simulink model "Demo_MostImportant_cs"  (R2014b)
settings: Solver=FixedStepDiscrete  SolverMode=SingleTasking  StartTime=0.0  StopTime=18  FixedStep=1/20  RelTol=1e-3
PreLoadFcn:
  | mbxruntime.callbacks.PreLoadFcn(bdroot);
  | check_NUTS_defined
  | model_closed = 0;
  | assignin('base',['model_closed_' bdroot],false);
PostLoadFcn:
  | mbxruntime.callbacks.PostLoadFcn(bdroot);
InitFcn:
  | mbxruntime.callbacks.InitFcn(bdroot);
StartFcn:
  | mbxruntime.callbacks.StartFcn(bdroot);
StopFcn:
  | mbxruntime.callbacks.StopFcn(bdroot);;
  | 
model workspace: external: MAT-File .\Demo_MostImportant_cs_hws.mat (data not in the file)
undefined symbols (not defined in the file or in its folder): mbxruntime, tabledata
undefined symbols (not defined in the file): Demo_MostImportant_cs_05200168a21c2533, Demo_MostImportant_cs_094a97935dc182a0, Demo_MostImportant_cs_0f0a9e0d54ccafda, Demo_MostImportant_cs_0fd3352235f3d862, Demo_MostImportant_cs_143c6c4f39bdc546, Demo_MostImportant_cs_20660bde6631f89a, Demo_MostImportant_cs_22077597b1c7a4aa, Demo_MostImportant_cs_22569723bd476150, Demo_MostImportant_cs_25eb058b93ed81ed, Demo_MostImportant_cs_27ad505fd49d0562, Demo_MostImportant_cs_3388db03542917da, Demo_MostImportant_cs_3411dde5ae0dc98c, Demo_MostImportant_cs_365f965ea4b6cb52, Demo_MostImportant_cs_3bee97dace5a3f8a, Demo_MostImportant_cs_3d2ef73ad714ff29, Demo_MostImportant_cs_4312029ae1b23d3a, Demo_MostImportant_cs_431f249e57fff8cb, Demo_MostImportant_cs_437388c3dfd4518f, Demo_MostImportant_cs_439f7e889f94edbe, Demo_MostImportant_cs_44a44174db621f6d, Demo_MostImportant_cs_4a7f7efcfc625194, Demo_MostImportant_cs_4a85c22e4a955f8e, Demo_MostImportant_cs_4c0e276e17a8ce88, Demo_MostImportant_cs_4cf092a47043b63b, Demo_MostImportant_cs_528dc6b548c718e3, Demo_MostImportant_cs_554a5828426d1258, Demo_MostImportant_cs_5a7163d13d0d3a72, Demo_MostImportant_cs_5d58a9d5d373adee, Demo_MostImportant_cs_60fd2791e6a88e66, Demo_MostImportant_cs_62ee6b3874c5d210, Demo_MostImportant_cs_63cb394815d07d4b, Demo_MostImportant_cs_660ed07c6769932e, Demo_MostImportant_cs_704620a5d39b7df9, Demo_MostImportant_cs_715ca1aaa17d3e85, Demo_MostImportant_cs_72b0848bf20979d6, Demo_MostImportant_cs_786125b10b06ee8f, Demo_MostImportant_cs_7e81a3b41a2b3c89, Demo_MostImportant_cs_81a32c4ed1a9050c, Demo_MostImportant_cs_883a94dece8b903d, Demo_MostImportant_cs_90ff3a0811121d4c, Demo_MostImportant_cs_912cf0a5d0300393, Demo_MostImportant_cs_99d08ec3ace083e5, Demo_MostImportant_cs_9be8f6a6d15b97ae, Demo_MostImportant_cs_a1434df4461c57cd, Demo_MostImportant_cs_a9807fe959845dbd, Demo_MostImportant_cs_ad42817c2f688b9e, Demo_MostImportant_cs_Audi_A8_2_Path_pathUniqueID, Demo_MostImportant_cs_b5f63321977d4686, Demo_MostImportant_cs_bae02335aafbc09b, Demo_MostImportant_cs_bdb138340502b82e, Demo_MostImportant_cs_be891ccddc71916a, Demo_MostImportant_cs_BMW_X5_1_Path_pathUniqueID, Demo_MostImportant_cs_BMW_X5_2_Path_pathUniqueID, Demo_MostImportant_cs_c0dcb6f642224268, Demo_MostImportant_cs_c311fdddc66ce1e1, Demo_MostImportant_cs_c34fad1f7dbabd44, Demo_MostImportant_cs_c3ed80f4b140c4cf, Demo_MostImportant_cs_c71d57cd5d2ef8b2, Demo_MostImportant_cs_Citroen_C3_2_Path_pathUniqueID, Demo_MostImportant_cs_d6fc18532502b855 ... (+12)
libraries: PreScanSimulinkLibrary x20, simulink x16, PreScanUsefulBlocks x1
(part 4 of 7)

== system Demo_MostImportant_cs/VISUColorRegion_Exterior_Audi_A8_1 ==
  VISUColorRegion_Exterior_Audi_A8_1 : Inport  Tag=inport/ColorRegion  OutDataTypeStr=Bus: PRESCAN_COLOR_DATA  PortDimensions=1  SampleTime=1/20  BusOutputAsStruct=on
  Actuator : S-Function  FunctionName=sfun_ColorActuator  Parameters=mbxruntime.parameters.convert(UniqueID), mbxruntime.parameters.convert(WorldModelSubPath),tabledata, TimeStep  EnableBusSupport=off  mask(PreScan Sink Block: VisuTextureColor){UniqueID=49, WorldModelSubPath=/recolorRegion:name=Exterior/targetColor, TimeStep=1/20}
      mask prompts: UniqueID "Parent Unique Identifier (auto-generated)"; WorldModelSubPath "WM SubPath(auto-generated)"; TimeStep "Simulink time step"
      mask help:
      | The VisuTextureColor block provides a way to adapt the color of a vehicle.
      |
      | For more information, please click Help.
      mask init:
      | [tabledata] = mbxruntime.parameters.table(UniqueID,WorldModelSubPath);
      mask Help: eval('openHelp(230)')
      mask Display: image(imread('TextureColor.png'))
  wires:
  VISUColorRegion_Exterior_Audi_A8_1/1 -> Actuator/1

== system Demo_MostImportant_cs/VISUColorRegion_Exterior_Audi_A8_2 ==
  VISUColorRegion_Exterior_Audi_A8_2 : Inport  Tag=inport/ColorRegion  OutDataTypeStr=Bus: PRESCAN_COLOR_DATA  PortDimensions=1  SampleTime=1/20  BusOutputAsStruct=on
  Actuator : S-Function  FunctionName=sfun_ColorActuator  Parameters=mbxruntime.parameters.convert(UniqueID), mbxruntime.parameters.convert(WorldModelSubPath),tabledata, TimeStep  EnableBusSupport=off  mask(PreScan Sink Block: VisuTextureColor){UniqueID=107, WorldModelSubPath=/recolorRegion:name=Exterior/targetColor, TimeStep=1/20}
      mask prompts: UniqueID "Parent Unique Identifier (auto-generated)"; WorldModelSubPath "WM SubPath(auto-generated)"; TimeStep "Simulink time step"
      mask help:
      | The VisuTextureColor block provides a way to adapt the color of a vehicle.
      |
      | For more information, please click Help.
      mask init:
      | [tabledata] = mbxruntime.parameters.table(UniqueID,WorldModelSubPath);
      mask Help: eval('openHelp(230)')
      mask Display: image(imread('TextureColor.png'))
  wires:
  VISUColorRegion_Exterior_Audi_A8_2/1 -> Actuator/1

== system Demo_MostImportant_cs/VISUColorRegion_Exterior_Audi_A8_3 ==
  VISUColorRegion_Exterior_Audi_A8_3 : Inport  Tag=inport/ColorRegion  OutDataTypeStr=Bus: PRESCAN_COLOR_DATA  PortDimensions=1  SampleTime=1/20  BusOutputAsStruct=on
  Actuator : S-Function  FunctionName=sfun_ColorActuator  Parameters=mbxruntime.parameters.convert(UniqueID), mbxruntime.parameters.convert(WorldModelSubPath),tabledata, TimeStep  EnableBusSupport=off  mask(PreScan Sink Block: VisuTextureColor){UniqueID=143, WorldModelSubPath=/recolorRegion:name=Exterior/targetColor, TimeStep=1/20}
      mask prompts: UniqueID "Parent Unique Identifier (auto-generated)"; WorldModelSubPath "WM SubPath(auto-generated)"; TimeStep "Simulink time step"
      mask help:
      | The VisuTextureColor block provides a way to adapt the color of a vehicle.
      |
      | For more information, please click Help.
      mask init:
      | [tabledata] = mbxruntime.parameters.table(UniqueID,WorldModelSubPath);
      mask Help: eval('openHelp(230)')
      mask Display: image(imread('TextureColor.png'))
  wires:
  VISUColorRegion_Exterior_Audi_A8_3/1 -> Actuator/1

== system Demo_MostImportant_cs/VISUColorRegion_Exterior_BMW_X5_1 ==
  VISUColorRegion_Exterior_BMW_X5_1 : Inport  Tag=inport/ColorRegion  OutDataTypeStr=Bus: PRESCAN_COLOR_DATA  PortDimensions=1  SampleTime=1/20  BusOutputAsStruct=on
  Actuator : S-Function  FunctionName=sfun_ColorActuator  Parameters=mbxruntime.parameters.convert(UniqueID), mbxruntime.parameters.convert(WorldModelSubPath),tabledata, TimeStep  EnableBusSupport=off  mask(PreScan Sink Block: VisuTextureColor){UniqueID=19, WorldModelSubPath=/recolorRegion:name=Exterior/targetColor, TimeStep=1/20}
      mask prompts: UniqueID "Parent Unique Identifier (auto-generated)"; WorldModelSubPath "WM SubPath(auto-generated)"; TimeStep "Simulink time step"
      mask help:
      | The VisuTextureColor block provides a way to adapt the color of a vehicle.
      |
      | For more information, please click Help.
      mask init:
      | [tabledata] = mbxruntime.parameters.table(UniqueID,WorldModelSubPath);
      mask Help: eval('openHelp(230)')
      mask Display: image(imread('TextureColor.png'))
  wires:
  VISUColorRegion_Exterior_BMW_X5_1/1 -> Actuator/1

== system Demo_MostImportant_cs/VISUColorRegion_Exterior_BMW_X5_2 ==
  VISUColorRegion_Exterior_BMW_X5_2 : Inport  Tag=inport/ColorRegion  OutDataTypeStr=Bus: PRESCAN_COLOR_DATA  PortDimensions=1  SampleTime=1/20  BusOutputAsStruct=on
  Actuator : S-Function  FunctionName=sfun_ColorActuator  Parameters=mbxruntime.parameters.convert(UniqueID), mbxruntime.parameters.convert(WorldModelSubPath),tabledata, TimeStep  EnableBusSupport=off  mask(PreScan Sink Block: VisuTextureColor){UniqueID=111, WorldModelSubPath=/recolorRegion:name=Exterior/targetColor, TimeStep=1/20}
      mask prompts: UniqueID "Parent Unique Identifier (auto-generated)"; WorldModelSubPath "WM SubPath(auto-generated)"; TimeStep "Simulink time step"
      mask help:
      | The VisuTextureColor block provides a way to adapt the color of a vehicle.
      |
      | For more information, please click Help.
      mask init:
      | [tabledata] = mbxruntime.parameters.table(UniqueID,WorldModelSubPath);
      mask Help: eval('openHelp(230)')
      mask Display: image(imread('TextureColor.png'))
  wires:
  VISUColorRegion_Exterior_BMW_X5_2/1 -> Actuator/1

== system Demo_MostImportant_cs/VISUColorRegion_Exterior_Citroen_C3_1 ==
  VISUColorRegion_Exterior_Citroen_C3_1 : Inport  Tag=inport/ColorRegion  OutDataTypeStr=Bus: PRESCAN_COLOR_DATA  PortDimensions=1  SampleTime=1/20  BusOutputAsStruct=on
  Actuator : S-Function  FunctionName=sfun_ColorActuator  Parameters=mbxruntime.parameters.convert(UniqueID), mbxruntime.parameters.convert(WorldModelSubPath),tabledata, TimeStep  EnableBusSupport=off  mask(PreScan Sink Block: VisuTextureColor){UniqueID=45, WorldModelSubPath=/recolorRegion:name=Exterior/targetColor, TimeStep=1/20}
      mask prompts: UniqueID "Parent Unique Identifier (auto-generated)"; WorldModelSubPath "WM SubPath(auto-generated)"; TimeStep "Simulink time step"
      mask help:
      | The VisuTextureColor block provides a way to adapt the color of a vehicle.
      |
      | For more information, please click Help.
      mask init:
      | [tabledata] = mbxruntime.parameters.table(UniqueID,WorldModelSubPath);
      mask Help: eval('openHelp(230)')
      mask Display: image(imread('TextureColor.png'))
  wires:
  VISUColorRegion_Exterior_Citroen_C3_1/1 -> Actuator/1

== system Demo_MostImportant_cs/VISUColorRegion_Exterior_Citroen_C3_2 ==
  VISUColorRegion_Exterior_Citroen_C3_2 : Inport  Tag=inport/ColorRegion  OutDataTypeStr=Bus: PRESCAN_COLOR_DATA  PortDimensions=1  SampleTime=1/20  BusOutputAsStruct=on
  Actuator : S-Function  FunctionName=sfun_ColorActuator  Parameters=mbxruntime.parameters.convert(UniqueID), mbxruntime.parameters.convert(WorldModelSubPath),tabledata, TimeStep  EnableBusSupport=off  mask(PreScan Sink Block: VisuTextureColor){UniqueID=117, WorldModelSubPath=/recolorRegion:name=Exterior/targetColor, TimeStep=1/20}
      mask prompts: UniqueID "Parent Unique Identifier (auto-generated)"; WorldModelSubPath "WM SubPath(auto-generated)"; TimeStep "Simulink time step"
      mask help:
      | The VisuTextureColor block provides a way to adapt the color of a vehicle.
      |
      | For more information, please click Help.
      mask init:
      | [tabledata] = mbxruntime.parameters.table(UniqueID,WorldModelSubPath);
      mask Help: eval('openHelp(230)')
      mask Display: image(imread('TextureColor.png'))
  wires:
  VISUColorRegion_Exterior_Citroen_C3_2/1 -> Actuator/1

== system Demo_MostImportant_cs/VISUColorRegion_Exterior_Citroen_C3_3 ==
  VISUColorRegion_Exterior_Citroen_C3_3 : Inport  Tag=inport/ColorRegion  OutDataTypeStr=Bus: PRESCAN_COLOR_DATA  PortDimensions=1  SampleTime=1/20  BusOutputAsStruct=on
  Actuator : S-Function  FunctionName=sfun_ColorActuator  Parameters=mbxruntime.parameters.convert(UniqueID), mbxruntime.parameters.convert(WorldModelSubPath),tabledata, TimeStep  EnableBusSupport=off  mask(PreScan Sink Block: VisuTextureColor){UniqueID=139, WorldModelSubPath=/recolorRegion:name=Exterior/targetColor, TimeStep=1/20}
      mask prompts: UniqueID "Parent Unique Identifier (auto-generated)"; WorldModelSubPath "WM SubPath(auto-generated)"; TimeStep "Simulink time step"
      mask help:
      | The VisuTextureColor block provides a way to adapt the color of a vehicle.
      |
      | For more information, please click Help.
      mask init:
      | [tabledata] = mbxruntime.parameters.table(UniqueID,WorldModelSubPath);
      mask Help: eval('openHelp(230)')
      mask Display: image(imread('TextureColor.png'))
  wires:
  VISUColorRegion_Exterior_Citroen_C3_3/1 -> Actuator/1

== system Demo_MostImportant_cs/VISUColorRegion_Exterior_Citroen_C3_4 ==
  VISUColorRegion_Exterior_Citroen_C3_4 : Inport  Tag=inport/ColorRegion  OutDataTypeStr=Bus: PRESCAN_COLOR_DATA  PortDimensions=1  SampleTime=1/20  BusOutputAsStruct=on
  Actuator : S-Function  FunctionName=sfun_ColorActuator  Parameters=mbxruntime.parameters.convert(UniqueID), mbxruntime.parameters.convert(WorldModelSubPath),tabledata, TimeStep  EnableBusSupport=off  mask(PreScan Sink Block: VisuTextureColor){UniqueID=140, WorldModelSubPath=/recolorRegion:name=Exterior/targetColor, TimeStep=1/20}
      mask prompts: UniqueID "Parent Unique Identifier (auto-generated)"; WorldModelSubPath "WM SubPath(auto-generated)"; TimeStep "Simulink time step"
      mask help:
      | The VisuTextureColor block provides a way to adapt the color of a vehicle.
      |
      | For more information, please click Help.
      mask init:
      | [tabledata] = mbxruntime.parameters.table(UniqueID,WorldModelSubPath);
      mask Help: eval('openHelp(230)')
      mask Display: image(imread('TextureColor.png'))
  wires:
  VISUColorRegion_Exterior_Citroen_C3_4/1 -> Actuator/1

== system Demo_MostImportant_cs/VISUColorRegion_Exterior_Toyota_Previa_1 ==
  VISUColorRegion_Exterior_Toyota_Previa_1 : Inport  Tag=inport/ColorRegion  OutDataTypeStr=Bus: PRESCAN_COLOR_DATA  PortDimensions=1  SampleTime=1/20  BusOutputAsStruct=on
  Actuator : S-Function  FunctionName=sfun_ColorActuator  Parameters=mbxruntime.parameters.convert(UniqueID), mbxruntime.parameters.convert(WorldModelSubPath),tabledata, TimeStep  EnableBusSupport=off  mask(PreScan Sink Block: VisuTextureColor){UniqueID=15, WorldModelSubPath=/recolorRegion:name=Exterior/targetColor, TimeStep=1/20}
      mask prompts: UniqueID "Parent Unique Identifier (auto-generated)"; WorldModelSubPath "WM SubPath(auto-generated)"; TimeStep "Simulink time step"
      mask help:
      | The VisuTextureColor block provides a way to adapt the color of a vehicle.
      |
      | For more information, please click Help.
      mask init:
      | [tabledata] = mbxruntime.parameters.table(UniqueID,WorldModelSubPath);
      mask Help: eval('openHelp(230)')
      mask Display: image(imread('TextureColor.png'))
  wires:
  VISUColorRegion_Exterior_Toyota_Previa_1/1 -> Actuator/1

== system Demo_MostImportant_cs/VISUColorRegion_Exterior_Toyota_Previa_2 ==
  VISUColorRegion_Exterior_Toyota_Previa_2 : Inport  Tag=inport/ColorRegion  OutDataTypeStr=Bus: PRESCAN_COLOR_DATA  PortDimensions=1  SampleTime=1/20  BusOutputAsStruct=on
  Actuator : S-Function  FunctionName=sfun_ColorActuator  Parameters=mbxruntime.parameters.convert(UniqueID), mbxruntime.parameters.convert(WorldModelSubPath),tabledata, TimeStep  EnableBusSupport=off  mask(PreScan Sink Block: VisuTextureColor){UniqueID=99, WorldModelSubPath=/recolorRegion:name=Exterior/targetColor, TimeStep=1/20}
      mask prompts: UniqueID "Parent Unique Identifier (auto-generated)"; WorldModelSubPath "WM SubPath(auto-generated)"; TimeStep "Simulink time step"
      mask help:
      | The VisuTextureColor block provides a way to adapt the color of a vehicle.
      |
      | For more information, please click Help.
      mask init:
      | [tabledata] = mbxruntime.parameters.table(UniqueID,WorldModelSubPath);
      mask Help: eval('openHelp(230)')
      mask Display: image(imread('TextureColor.png'))
  wires:
  VISUColorRegion_Exterior_Toyota_Previa_2/1 -> Actuator/1

== system Demo_MostImportant_cs/VISUColorRegion_Exterior_Toyota_Previa_3 ==
  VISUColorRegion_Exterior_Toyota_Previa_3 : Inport  Tag=inport/ColorRegion  OutDataTypeStr=Bus: PRESCAN_COLOR_DATA  PortDimensions=1  SampleTime=1/20  BusOutputAsStruct=on
  Actuator : S-Function  FunctionName=sfun_ColorActuator  Parameters=mbxruntime.parameters.convert(UniqueID), mbxruntime.parameters.convert(WorldModelSubPath),tabledata, TimeStep  EnableBusSupport=off  mask(PreScan Sink Block: VisuTextureColor){UniqueID=123, WorldModelSubPath=/recolorRegion:name=Exterior/targetColor, TimeStep=1/20}
      mask prompts: UniqueID "Parent Unique Identifier (auto-generated)"; WorldModelSubPath "WM SubPath(auto-generated)"; TimeStep "Simulink time step"
      mask help:
      | The VisuTextureColor block provides a way to adapt the color of a vehicle.
      |
      | For more information, please click Help.
      mask init:
      | [tabledata] = mbxruntime.parameters.table(UniqueID,WorldModelSubPath);
      mask Help: eval('openHelp(230)')
      mask Display: image(imread('TextureColor.png'))
  wires:
  VISUColorRegion_Exterior_Toyota_Previa_3/1 -> Actuator/1

== system Demo_MostImportant_cs/VISUColorRegion_Exterior_Toyota_Previa_4 ==
  VISUColorRegion_Exterior_Toyota_Previa_4 : Inport  Tag=inport/ColorRegion  OutDataTypeStr=Bus: PRESCAN_COLOR_DATA  PortDimensions=1  SampleTime=1/20  BusOutputAsStruct=on
  Actuator : S-Function  FunctionName=sfun_ColorActuator  Parameters=mbxruntime.parameters.convert(UniqueID), mbxruntime.parameters.convert(WorldModelSubPath),tabledata, TimeStep  EnableBusSupport=off  mask(PreScan Sink Block: VisuTextureColor){UniqueID=141, WorldModelSubPath=/recolorRegion:name=Exterior/targetColor, TimeStep=1/20}
      mask prompts: UniqueID "Parent Unique Identifier (auto-generated)"; WorldModelSubPath "WM SubPath(auto-generated)"; TimeStep "Simulink time step"
      mask help:
      | The VisuTextureColor block provides a way to adapt the color of a vehicle.
      |
      | For more information, please click Help.
      mask init:
      | [tabledata] = mbxruntime.parameters.table(UniqueID,WorldModelSubPath);
      mask Help: eval('openHelp(230)')
      mask Display: image(imread('TextureColor.png'))
  wires:
  VISUColorRegion_Exterior_Toyota_Previa_4/1 -> Actuator/1

== system Demo_MostImportant_cs/VISUColorRegion_Exterior_Toyota_Yaris_1 ==
  VISUColorRegion_Exterior_Toyota_Yaris_1 : Inport  Tag=inport/ColorRegion  OutDataTypeStr=Bus: PRESCAN_COLOR_DATA  PortDimensions=1  SampleTime=1/20  BusOutputAsStruct=on
  Actuator : S-Function  FunctionName=sfun_ColorActuator  Parameters=mbxruntime.parameters.convert(UniqueID), mbxruntime.parameters.convert(WorldModelSubPath),tabledata, TimeStep  EnableBusSupport=off  mask(PreScan Sink Block: VisuTextureColor){UniqueID=46, WorldModelSubPath=/recolorRegion:name=Exterior/targetColor, TimeStep=1/20}
      mask prompts: UniqueID "Parent Unique Identifier (auto-generated)"; WorldModelSubPath "WM SubPath(auto-generated)"; TimeStep "Simulink time step"
      mask help:
      | The VisuTextureColor block provides a way to adapt the color of a vehicle.
      |
      | For more information, please click Help.
      mask init:
      | [tabledata] = mbxruntime.parameters.table(UniqueID,WorldModelSubPath);
      mask Help: eval('openHelp(230)')
      mask Display: image(imread('TextureColor.png'))
  wires:
  VISUColorRegion_Exterior_Toyota_Yaris_1/1 -> Actuator/1

== system Demo_MostImportant_cs/VISUColorRegion_Exterior_Toyota_Yaris_2 ==
  VISUColorRegion_Exterior_Toyota_Yaris_2 : Inport  Tag=inport/ColorRegion  OutDataTypeStr=Bus: PRESCAN_COLOR_DATA  PortDimensions=1  SampleTime=1/20  BusOutputAsStruct=on
  Actuator : S-Function  FunctionName=sfun_ColorActuator  Parameters=mbxruntime.parameters.convert(UniqueID), mbxruntime.parameters.convert(WorldModelSubPath),tabledata, TimeStep  EnableBusSupport=off  mask(PreScan Sink Block: VisuTextureColor){UniqueID=142, WorldModelSubPath=/recolorRegion:name=Exterior/targetColor, TimeStep=1/20}
      mask prompts: UniqueID "Parent Unique Identifier (auto-generated)"; WorldModelSubPath "WM SubPath(auto-generated)"; TimeStep "Simulink time step"
      mask help:
      | The VisuTextureColor block provides a way to adapt the color of a vehicle.
      |
      | For more information, please click Help.
      mask init:
      | [tabledata] = mbxruntime.parameters.table(UniqueID,WorldModelSubPath);
      mask Help: eval('openHelp(230)')
      mask Display: image(imread('TextureColor.png'))
  wires:
  VISUColorRegion_Exterior_Toyota_Yaris_2/1 -> Actuator/1

== system Demo_MostImportant_cs/Audi_A8_1/Dynamics_Empty ==
  note: For state mode 'Dynamic' positions
      | are not taken into account, as they
      | are computed by integrating velocity.
      | Click annotation for Help.
  Ground_{1..9} (9 alike) : Ground
  MuxState : Subsystem  Tag=mux/State  mask(Empty Dynamics State Block){positioningmode=on, TimeStep=1/20}
      mask prompts: positioningmode "Positioning Mode"; TimeStep "Auto Assigned: Time Step [s]"
      mask help:
      | Build the state of an actor based on user input.
      | The user can either use positioning mode or dynamics mode.
      | - When using positioning mode the position and orientation of the actor are set directly based on the input. Expected input is relative to the initial position and orientation of the actor. It's also possible to specify the velocity of the actor, though this input isn't used, only passed on.
      | - When using dynamics mode the position input is ignored. Expected input is velocity and orientation. The velocity is relative the current orientation of the actor, while orientation is relative to its initial orientation. The position of the actor is calculated based on the velocity and orientation given.
      settings: DeleteFcn=PreScanBlockDeleteFcn;
  STATE_Audi_A8_1 : Subsystem  Tag=mux/StatePort  Priority=0  LoadFcn=load PrescanStateActuatorData  mask(PreScan Sink Block: State){x0=Demo_MostImportant_cs_df769faa31fd9ead, y0=Demo_MostImportant_cs_f67437bd412fea32, z0=Demo_MostImportant_cs_f04d43c825bf3ceb, Roll0=Demo_MostImportant_cs_3411dde5ae0dc98c, Pitch0=Demo_MostImportant_cs_5d58a9d5d373adee, Yaw0=Demo_MostImportant_cs_554a5828426d1258, TimeStep=1/20}
      mask prompts: x0 "Ini x-position VEHICLE wrt GLOBAL axis system [m]"; y0 "Ini y-position VEHICLE wrt GLOBAL axis system [m]"; z0 "Ini z-position VEHICLE wrt GLOBAL axis system [m]"; Roll0 "Ini roll-angle BODY wrt VEHICLE axis system [deg]"; Pitch0 "Ini pitch-angle BODY wrt VEHICLE axis system [deg]"; Yaw0 "Ini yaw-angle VEHICLE wrt GLOBAL axis system [deg]"; TimeStep "Auto-Assigned: Upload Period [s]"
      mask help:
      | The Actor State contains a vector signal of size (9x1), containing the following signals:
      |
      | -  Position                  (x,y,z)                                     [m]
      | -  Velocity                  (vx,vy,vz)                               [m/s]
      | -  Angles                    (Roll, Pitch, Yaw)                   [rad]
      |
      | The Actor state is defined in the global axis system.
      | The state is superponed on the Initial position defined in the GUI.
      |
      | For more information, please click Help.
      settings: DeleteFcn=PreScanBlockDeleteFcn;
      mask Help: eval('openHelp(222)')
      mask Display: image(imread('State.png'))
  State : Outport  Tag=outport/StateOutport  SampleTime=1/20
  wires:
  MuxState/1(state) -> STATE_Audi_A8_1/1(State)
  STATE_Audi_A8_1/1(StateBus) -> State/1
  Ground_1/1 -> MuxState/1(x [m])
  Ground_2/1 -> MuxState/2(y [m])
  Ground_3/1 -> MuxState/3(z [m])
  Ground_4/1 -> MuxState/4(dx [m/s])
  Ground_5/1 -> MuxState/5(dy [m/s])
  Ground_6/1 -> MuxState/6(dz [m/s])
  Ground_7/1 -> MuxState/7(R [rad])
  Ground_8/1 -> MuxState/8(P [rad])
  Ground_9/1 -> MuxState/9(Y [rad])

== system Demo_MostImportant_cs/Audi_A8_1/SELF_Demux ==
  SELF : Inport  OutDataTypeStr=Bus: PRESCAN_SELFSENSORDATA
  Bus Selector : BusSelector  OutputSignals=PositionX,PositionY,PositionZ,OrientationRoll,OrientationPitch,OrientationYaw,Velocity,Yaw_rate,Lat,Long,Alt
  Demux2 : Demux  Outputs=3
  Gain : Gain  Gain=180/pi
  Gain1 : Gain  Gain=180/pi
  Vector Concatenate1 : Concatenate  NumInputs=3
  compas converter : Subsystem
  x [m] : Outport
  y [m] : Outport  Port=2
  z [m] : Outport  Port=3
  rotx [deg] : Outport  Port=4
  roty [deg] : Outport  Port=5
  rotz [deg] : Outport  Port=6
  GPS lat [deg] : Outport  Port=7
  GPS long [deg] : Outport  Port=8
  GPS alt [m] : Outport  Port=9
  velocity [m/s] : Outport  Port=10
  heading [deg] : Outport  Port=11
  yaw rate [deg/s] : Outport  Port=12
  wires:
  Bus Selector/11 -> GPS alt [m]/1  "<Alt>"
  Bus Selector/10 -> GPS long [deg]/1  "<Long>"
  Bus Selector/9 -> GPS lat [deg]/1  "<Lat>"
  Bus Selector/8 -> Gain1/1  "<Yaw_rate>"
  Bus Selector/7 -> velocity [m/s]/1  "<Velocity>"
  Bus Selector/6 -> compas converter/1(rotz [rad]), Vector Concatenate1/3  "<OrientationYaw>"
  Bus Selector/5 -> Vector Concatenate1/2  "<OrientationPitch>"
  Bus Selector/4 -> Vector Concatenate1/1  "<OrientationRoll>"
  Vector Concatenate1/1 -> Gain/1
  Bus Selector/3 -> z [m]/1  "<PositionZ>"
  Bus Selector/2 -> y [m]/1  "<PositionY>"
  Bus Selector/1 -> x [m]/1  "<PositionX>"
  SELF/1 -> Bus Selector/1
  Gain/1 -> Demux2/1
  Demux2/1 -> rotx [deg]/1
  Demux2/2 -> roty [deg]/1
  Demux2/3 -> rotz [deg]/1
  compas converter/1(heading [deg]) -> heading [deg]/1
  Gain1/1 -> yaw rate [deg/s]/1

== system Demo_MostImportant_cs/Audi_A8_1/VISUColorRegion_Exterior_Mux ==
  RGB [-,-,-] : Inport
  Bus Creator : BusCreator  OutDataTypeStr=Bus: PRESCAN_COLOR_DATA  NonVirtualBus=on
  Constant : Constant  Value=255  OutDataTypeStr=uint8
  Data Type Conversion : DataTypeConversion  OutDataTypeStr=uint8
  Data Type Conversion1 : DataTypeConversion  OutDataTypeStr=uint8
  Data Type Conversion2 : DataTypeConversion  OutDataTypeStr=uint8
  Demux : Demux  Outputs=3
  ColorRegion : Outport  OutDataTypeStr=Bus: PRESCAN_COLOR_DATA  PortDimensions=1
  wires:
  Constant/1 -> Bus Creator/4  "A"
  Data Type Conversion2/1 -> Bus Creator/3  "B"
  Data Type Conversion1/1 -> Bus Creator/2  "G"
  Data Type Conversion/1 -> Bus Creator/1  "R"
  Demux/3 -> Data Type Conversion2/1  "B"
  Demux/2 -> Data Type Conversion1/1  "G"
  Demux/1 -> Data Type Conversion/1  "R"
  RGB [-,-,-]/1 -> Demux/1
  Bus Creator/1 -> ColorRegion/1

== system Demo_MostImportant_cs/Audi_A8_1/color_changing_logic ==
  Index_order : Inport
  Compare To Constant : simulink/Logic and Bit Operations/Compare To Constant  relop=<=  const=3  OutDataTypeStr=uint8  ZeroCross=off
  Multiport Switch : MultiPortSwitch  DataPortOrder=Zero-based contiguous  Inputs=4  zeroidx=on
  Product : Product  RndMeth=Zero
  TextureColor1 : Constant  Tag=TextureColor  Value="[255 0  0]"
  TextureColor2 : Constant  Tag=TextureColor  Value="[211  211  211]"
  TextureColor3 : Constant  Tag=TextureColor  Value=[255 128 0]
  TextureColor4 : Constant  Tag=TextureColor  Value=[255 255 55]
  RGB : Outport
  wires:
  TextureColor2/1 -> Multiport Switch/2  "L21"
  TextureColor1/1 -> Multiport Switch/3  "L21"
  TextureColor3/1 -> Multiport Switch/4
  Compare To Constant/1 -> Product/2
  Index_order/1 -> Product/1, Compare To Constant/1
  Product/1 -> Multiport Switch/1
  Multiport Switch/1 -> RGB/1  "L47"
  TextureColor4/1 -> Multiport Switch/5

== system Demo_MostImportant_cs/Audi_A8_2/SELF_Demux ==
  SELF : Inport  OutDataTypeStr=Bus: PRESCAN_SELFSENSORDATA
  Bus Selector : BusSelector  OutputSignals=PositionX,PositionY,PositionZ,OrientationRoll,OrientationPitch,OrientationYaw,Velocity,Yaw_rate,Lat,Long,Alt
  Demux2 : Demux  Outputs=3
  Gain : Gain  Gain=180/pi
  Gain1 : Gain  Gain=180/pi
  Vector Concatenate1 : Concatenate  NumInputs=3
  compas converter : Subsystem
  x [m] : Outport
  y [m] : Outport  Port=2
  z [m] : Outport  Port=3
  rotx [deg] : Outport  Port=4
  roty [deg] : Outport  Port=5
  rotz [deg] : Outport  Port=6
  GPS lat [deg] : Outport  Port=7
  GPS long [deg] : Outport  Port=8
  GPS alt [m] : Outport  Port=9
  velocity [m/s] : Outport  Port=10
  heading [deg] : Outport  Port=11
  yaw rate [deg/s] : Outport  Port=12
  wires:
  Bus Selector/11 -> GPS alt [m]/1  "<Alt>"
  Bus Selector/10 -> GPS long [deg]/1  "<Long>"
  Bus Selector/9 -> GPS lat [deg]/1  "<Lat>"
  Bus Selector/8 -> Gain1/1  "<Yaw_rate>"
  Bus Selector/7 -> velocity [m/s]/1  "<Velocity>"
  Bus Selector/6 -> compas converter/1(rotz [rad]), Vector Concatenate1/3  "<OrientationYaw>"
  Bus Selector/5 -> Vector Concatenate1/2  "<OrientationPitch>"
  Bus Selector/4 -> Vector Concatenate1/1  "<OrientationRoll>"
  Vector Concatenate1/1 -> Gain/1
  Bus Selector/3 -> z [m]/1  "<PositionZ>"
  Bus Selector/2 -> y [m]/1  "<PositionY>"
  Bus Selector/1 -> x [m]/1  "<PositionX>"
  SELF/1 -> Bus Selector/1
  Gain/1 -> Demux2/1
  Demux2/1 -> rotx [deg]/1
  Demux2/2 -> roty [deg]/1
  Demux2/3 -> rotz [deg]/1
  compas converter/1(heading [deg]) -> heading [deg]/1
  Gain1/1 -> yaw rate [deg/s]/1

== system Demo_MostImportant_cs/Audi_A8_2/VISUColorRegion_Exterior_Mux ==
  RGB [-,-,-] : Inport
  Bus Creator : BusCreator  OutDataTypeStr=Bus: PRESCAN_COLOR_DATA  NonVirtualBus=on
  Constant : Constant  Value=255  OutDataTypeStr=uint8
  Data Type Conversion : DataTypeConversion  OutDataTypeStr=uint8
  Data Type Conversion1 : DataTypeConversion  OutDataTypeStr=uint8
  Data Type Conversion2 : DataTypeConversion  OutDataTypeStr=uint8
  Demux : Demux  Outputs=3
  ColorRegion : Outport  OutDataTypeStr=Bus: PRESCAN_COLOR_DATA  PortDimensions=1
  wires:
  Constant/1 -> Bus Creator/4  "A"
  Data Type Conversion2/1 -> Bus Creator/3  "B"
  Data Type Conversion1/1 -> Bus Creator/2  "G"
  Data Type Conversion/1 -> Bus Creator/1  "R"
  Demux/3 -> Data Type Conversion2/1  "B"
  Demux/2 -> Data Type Conversion1/1  "G"
  Demux/1 -> Data Type Conversion/1  "R"
  RGB [-,-,-]/1 -> Demux/1
  Bus Creator/1 -> ColorRegion/1

== system Demo_MostImportant_cs/Audi_A8_2/color_changing_logic ==
  Index_order : Inport
  Compare To Constant : simulink/Logic and Bit Operations/Compare To Constant  relop=<=  const=3  OutDataTypeStr=uint8  ZeroCross=off
  Multiport Switch : MultiPortSwitch  DataPortOrder=Zero-based contiguous  Inputs=4  zeroidx=on
  Product : Product  RndMeth=Zero
  TextureColor1 : Constant  Tag=TextureColor  Value="[255 0  0]"
  TextureColor2 : Constant  Tag=TextureColor  Value="[211  211  211]"
  TextureColor3 : Constant  Tag=TextureColor  Value=[255 128 0]
  TextureColor4 : Constant  Tag=TextureColor  Value=[255 255 55]
  RGB : Outport
  wires:
  TextureColor2/1 -> Multiport Switch/2  "L21"
  TextureColor1/1 -> Multiport Switch/3  "L21"
  TextureColor3/1 -> Multiport Switch/4
  Compare To Constant/1 -> Product/2
  Index_order/1 -> Product/1, Compare To Constant/1
  Product/1 -> Multiport Switch/1
  Multiport Switch/1 -> RGB/1  "L47"
  TextureColor4/1 -> Multiport Switch/5

== system Demo_MostImportant_cs/Audi_A8_3/Dynamics_Empty ==
  note: For state mode 'Dynamic' positions
      | are not taken into account, as they
      | are computed by integrating velocity.
      | Click annotation for Help.
  Ground_{1..9} (9 alike) : Ground
  MuxState : Subsystem  Tag=mux/State  mask(Empty Dynamics State Block){positioningmode=on, TimeStep=1/20}
      mask prompts: positioningmode "Positioning Mode"; TimeStep "Auto Assigned: Time Step [s]"
      mask help:
      | Build the state of an actor based on user input.
      | The user can either use positioning mode or dynamics mode.
      | - When using positioning mode the position and orientation of the actor are set directly based on the input. Expected input is relative to the initial position and orientation of the actor. It's also possible to specify the velocity of the actor, though this input isn't used, only passed on.
      | - When using dynamics mode the position input is ignored. Expected input is velocity and orientation. The velocity is relative the current orientation of the actor, while orientation is relative to its initial orientation. The position of the actor is calculated based on the velocity and orientation given.
      settings: DeleteFcn=PreScanBlockDeleteFcn;
  STATE_Audi_A8_3 : Subsystem  Tag=mux/StatePort  Priority=0  LoadFcn=load PrescanStateActuatorData  mask(PreScan Sink Block: State){x0=Demo_MostImportant_cs_ad42817c2f688b9e, y0=Demo_MostImportant_cs_4312029ae1b23d3a, z0=Demo_MostImportant_cs_a9807fe959845dbd, Roll0=Demo_MostImportant_cs_365f965ea4b6cb52, Pitch0=Demo_MostImportant_cs_3388db03542917da, Yaw0=Demo_MostImportant_cs_05200168a21c2533, TimeStep=1/20}
      mask prompts: x0 "Ini x-position VEHICLE wrt GLOBAL axis system [m]"; y0 "Ini y-position VEHICLE wrt GLOBAL axis system [m]"; z0 "Ini z-position VEHICLE wrt GLOBAL axis system [m]"; Roll0 "Ini roll-angle BODY wrt VEHICLE axis system [deg]"; Pitch0 "Ini pitch-angle BODY wrt VEHICLE axis system [deg]"; Yaw0 "Ini yaw-angle VEHICLE wrt GLOBAL axis system [deg]"; TimeStep "Auto-Assigned: Upload Period [s]"
      mask help:
      | The Actor State contains a vector signal of size (9x1), containing the following signals:
      |
      | -  Position                  (x,y,z)                                     [m]
      | -  Velocity                  (vx,vy,vz)                               [m/s]
      | -  Angles                    (Roll, Pitch, Yaw)                   [rad]
      |
      | The Actor state is defined in the global axis system.
      | The state is superponed on the Initial position defined in the GUI.
      |
      | For more information, please click Help.
      settings: DeleteFcn=PreScanBlockDeleteFcn;
      mask Help: eval('openHelp(222)')
      mask Display: image(imread('State.png'))
  State : Outport  Tag=outport/StateOutport  SampleTime=1/20
  wires:
  MuxState/1(state) -> STATE_Audi_A8_3/1(State)
  STATE_Audi_A8_3/1(StateBus) -> State/1
  Ground_1/1 -> MuxState/1(x [m])
  Ground_2/1 -> MuxState/2(y [m])
  Ground_3/1 -> MuxState/3(z [m])
  Ground_4/1 -> MuxState/4(dx [m/s])
  Ground_5/1 -> MuxState/5(dy [m/s])
  Ground_6/1 -> MuxState/6(dz [m/s])
  Ground_7/1 -> MuxState/7(R [rad])
  Ground_8/1 -> MuxState/8(P [rad])
  Ground_9/1 -> MuxState/9(Y [rad])

== system Demo_MostImportant_cs/Audi_A8_3/SELF_Demux ==
  SELF : Inport  OutDataTypeStr=Bus: PRESCAN_SELFSENSORDATA
  Bus Selector : BusSelector  OutputSignals=PositionX,PositionY,PositionZ,OrientationRoll,OrientationPitch,OrientationYaw,Velocity,Yaw_rate,Lat,Long,Alt
  Demux2 : Demux  Outputs=3
  Gain : Gain  Gain=180/pi
  Gain1 : Gain  Gain=180/pi
  Vector Concatenate1 : Concatenate  NumInputs=3
  compas converter : Subsystem
  x [m] : Outport
  y [m] : Outport  Port=2
  z [m] : Outport  Port=3
  rotx [deg] : Outport  Port=4
  roty [deg] : Outport  Port=5
  rotz [deg] : Outport  Port=6
  GPS lat [deg] : Outport  Port=7
  GPS long [deg] : Outport  Port=8
  GPS alt [m] : Outport  Port=9
  velocity [m/s] : Outport  Port=10
  heading [deg] : Outport  Port=11
  yaw rate [deg/s] : Outport  Port=12
  wires:
  Bus Selector/11 -> GPS alt [m]/1  "<Alt>"
  Bus Selector/10 -> GPS long [deg]/1  "<Long>"
  Bus Selector/9 -> GPS lat [deg]/1  "<Lat>"
  Bus Selector/8 -> Gain1/1  "<Yaw_rate>"
  Bus Selector/7 -> velocity [m/s]/1  "<Velocity>"
  Bus Selector/6 -> compas converter/1(rotz [rad]), Vector Concatenate1/3  "<OrientationYaw>"
  Bus Selector/5 -> Vector Concatenate1/2  "<OrientationPitch>"
  Bus Selector/4 -> Vector Concatenate1/1  "<OrientationRoll>"
  Vector Concatenate1/1 -> Gain/1
  Bus Selector/3 -> z [m]/1  "<PositionZ>"
  Bus Selector/2 -> y [m]/1  "<PositionY>"
  Bus Selector/1 -> x [m]/1  "<PositionX>"
  SELF/1 -> Bus Selector/1
  Gain/1 -> Demux2/1
  Demux2/1 -> rotx [deg]/1
  Demux2/2 -> roty [deg]/1
  Demux2/3 -> rotz [deg]/1
  compas converter/1(heading [deg]) -> heading [deg]/1
  Gain1/1 -> yaw rate [deg/s]/1

== system Demo_MostImportant_cs/Audi_A8_3/VISUColorRegion_Exterior_Mux ==
  RGB [-,-,-] : Inport
  Bus Creator : BusCreator  OutDataTypeStr=Bus: PRESCAN_COLOR_DATA  NonVirtualBus=on
  Constant : Constant  Value=255  OutDataTypeStr=uint8
  Data Type Conversion : DataTypeConversion  OutDataTypeStr=uint8
  Data Type Conversion1 : DataTypeConversion  OutDataTypeStr=uint8
  Data Type Conversion2 : DataTypeConversion  OutDataTypeStr=uint8
  Demux : Demux  Outputs=3
  ColorRegion : Outport  OutDataTypeStr=Bus: PRESCAN_COLOR_DATA  PortDimensions=1
  wires:
  Constant/1 -> Bus Creator/4  "A"
  Data Type Conversion2/1 -> Bus Creator/3  "B"
  Data Type Conversion1/1 -> Bus Creator/2  "G"
  Data Type Conversion/1 -> Bus Creator/1  "R"
  Demux/3 -> Data Type Conversion2/1  "B"
  Demux/2 -> Data Type Conversion1/1  "G"
  Demux/1 -> Data Type Conversion/1  "R"
  RGB [-,-,-]/1 -> Demux/1
  Bus Creator/1 -> ColorRegion/1

== system Demo_MostImportant_cs/Audi_A8_3/color_changing_logic ==
  Index_order : Inport
  Compare To Constant : simulink/Logic and Bit Operations/Compare To Constant  relop=<=  const=3  OutDataTypeStr=uint8  ZeroCross=off
  Multiport Switch : MultiPortSwitch  DataPortOrder=Zero-based contiguous  Inputs=4  zeroidx=on
  Product : Product  RndMeth=Zero
  TextureColor1 : Constant  Tag=TextureColor  Value="[255 0  0]"
  TextureColor2 : Constant  Tag=TextureColor  Value="[211  211  211]"
  TextureColor3 : Constant  Tag=TextureColor  Value=[255 128 0]
  TextureColor4 : Constant  Tag=TextureColor  Value=[255 255 55]
  RGB : Outport
  wires:
  TextureColor2/1 -> Multiport Switch/2  "L21"
  TextureColor1/1 -> Multiport Switch/3  "L21"
  TextureColor3/1 -> Multiport Switch/4
  Compare To Constant/1 -> Product/2
  Index_order/1 -> Product/1, Compare To Constant/1
  Product/1 -> Multiport Switch/1
  Multiport Switch/1 -> RGB/1  "L47"
  TextureColor4/1 -> Multiport Switch/5

== system Demo_MostImportant_cs/BMW_X5_1/SELF_Demux ==
  SELF : Inport  OutDataTypeStr=Bus: PRESCAN_SELFSENSORDATA
  Bus Selector : BusSelector  OutputSignals=PositionX,PositionY,PositionZ,OrientationRoll,OrientationPitch,OrientationYaw,Velocity,Yaw_rate,Lat,Long,Alt
  Demux2 : Demux  Outputs=3
  Gain : Gain  Gain=180/pi
  Gain1 : Gain  Gain=180/pi
  Vector Concatenate1 : Concatenate  NumInputs=3
  compas converter : Subsystem
  x [m] : Outport
  y [m] : Outport  Port=2
  z [m] : Outport  Port=3
  rotx [deg] : Outport  Port=4
  roty [deg] : Outport  Port=5
  rotz [deg] : Outport  Port=6
  GPS lat [deg] : Outport  Port=7
  GPS long [deg] : Outport  Port=8
  GPS alt [m] : Outport  Port=9
  velocity [m/s] : Outport  Port=10
  heading [deg] : Outport  Port=11
  yaw rate [deg/s] : Outport  Port=12
  wires:
  Bus Selector/11 -> GPS alt [m]/1  "<Alt>"
  Bus Selector/10 -> GPS long [deg]/1  "<Long>"
  Bus Selector/9 -> GPS lat [deg]/1  "<Lat>"
  Bus Selector/8 -> Gain1/1  "<Yaw_rate>"
  Bus Selector/7 -> velocity [m/s]/1  "<Velocity>"
  Bus Selector/6 -> compas converter/1(rotz [rad]), Vector Concatenate1/3  "<OrientationYaw>"
  Bus Selector/5 -> Vector Concatenate1/2  "<OrientationPitch>"
  Bus Selector/4 -> Vector Concatenate1/1  "<OrientationRoll>"
  Vector Concatenate1/1 -> Gain/1
  Bus Selector/3 -> z [m]/1  "<PositionZ>"
  Bus Selector/2 -> y [m]/1  "<PositionY>"
  Bus Selector/1 -> x [m]/1  "<PositionX>"
  SELF/1 -> Bus Selector/1
  Gain/1 -> Demux2/1
  Demux2/1 -> rotx [deg]/1
  Demux2/2 -> roty [deg]/1
  Demux2/3 -> rotz [deg]/1
  compas converter/1(heading [deg]) -> heading [deg]/1
  Gain1/1 -> yaw rate [deg/s]/1

== system Demo_MostImportant_cs/BMW_X5_1/VISUColorRegion_Exterior_Mux ==
  RGB [-,-,-] : Inport
  Bus Creator : BusCreator  OutDataTypeStr=Bus: PRESCAN_COLOR_DATA  NonVirtualBus=on
  Constant : Constant  Value=255  OutDataTypeStr=uint8
  Data Type Conversion : DataTypeConversion  OutDataTypeStr=uint8
  Data Type Conversion1 : DataTypeConversion  OutDataTypeStr=uint8
  Data Type Conversion2 : DataTypeConversion  OutDataTypeStr=uint8
  Demux : Demux  Outputs=3
  ColorRegion : Outport  OutDataTypeStr=Bus: PRESCAN_COLOR_DATA  PortDimensions=1
  wires:
  Constant/1 -> Bus Creator/4  "A"
  Data Type Conversion2/1 -> Bus Creator/3  "B"
  Data Type Conversion1/1 -> Bus Creator/2  "G"
  Data Type Conversion/1 -> Bus Creator/1  "R"
  Demux/3 -> Data Type Conversion2/1  "B"
  Demux/2 -> Data Type Conversion1/1  "G"
  Demux/1 -> Data Type Conversion/1  "R"
  RGB [-,-,-]/1 -> Demux/1
  Bus Creator/1 -> ColorRegion/1

== system Demo_MostImportant_cs/BMW_X5_1/color_changing_logic ==
  Index_order : Inport
  Compare To Constant : simulink/Logic and Bit Operations/Compare To Constant  relop=<=  const=3  OutDataTypeStr=uint8  ZeroCross=off
  Multiport Switch : MultiPortSwitch  DataPortOrder=Zero-based contiguous  Inputs=4  zeroidx=on
  Product : Product  RndMeth=Zero
  TextureColor1 : Constant  Tag=TextureColor  Value="[255 0  0]"
  TextureColor2 : Constant  Tag=TextureColor  Value="[211  211  211]"
  TextureColor3 : Constant  Tag=TextureColor  Value=[255 128 0]
  TextureColor4 : Constant  Tag=TextureColor  Value=[255 255 55]
  RGB : Outport
  wires:
  TextureColor2/1 -> Multiport Switch/2  "L21"
  TextureColor1/1 -> Multiport Switch/3  "L21"
  TextureColor3/1 -> Multiport Switch/4
  Compare To Constant/1 -> Product/2
  Index_order/1 -> Product/1, Compare To Constant/1
  Product/1 -> Multiport Switch/1
  Multiport Switch/1 -> RGB/1  "L47"
  TextureColor4/1 -> Multiport Switch/5

== system Demo_MostImportant_cs/BMW_X5_2/SELF_Demux ==
  SELF : Inport  OutDataTypeStr=Bus: PRESCAN_SELFSENSORDATA
  Bus Selector : BusSelector  OutputSignals=PositionX,PositionY,PositionZ,OrientationRoll,OrientationPitch,OrientationYaw,Velocity,Yaw_rate,Lat,Long,Alt
  Demux2 : Demux  Outputs=3
  Gain : Gain  Gain=180/pi
  Gain1 : Gain  Gain=180/pi
  Vector Concatenate1 : Concatenate  NumInputs=3
  compas converter : Subsystem
  x [m] : Outport
  y [m] : Outport  Port=2
  z [m] : Outport  Port=3
  rotx [deg] : Outport  Port=4
  roty [deg] : Outport  Port=5
  rotz [deg] : Outport  Port=6
  GPS lat [deg] : Outport  Port=7
  GPS long [deg] : Outport  Port=8
  GPS alt [m] : Outport  Port=9
  velocity [m/s] : Outport  Port=10
  heading [deg] : Outport  Port=11
  yaw rate [deg/s] : Outport  Port=12
  wires:
  Bus Selector/11 -> GPS alt [m]/1  "<Alt>"
  Bus Selector/10 -> GPS long [deg]/1  "<Long>"
  Bus Selector/9 -> GPS lat [deg]/1  "<Lat>"
  Bus Selector/8 -> Gain1/1  "<Yaw_rate>"
  Bus Selector/7 -> velocity [m/s]/1  "<Velocity>"
  Bus Selector/6 -> compas converter/1(rotz [rad]), Vector Concatenate1/3  "<OrientationYaw>"
  Bus Selector/5 -> Vector Concatenate1/2  "<OrientationPitch>"
  Bus Selector/4 -> Vector Concatenate1/1  "<OrientationRoll>"
  Vector Concatenate1/1 -> Gain/1
  Bus Selector/3 -> z [m]/1  "<PositionZ>"
  Bus Selector/2 -> y [m]/1  "<PositionY>"
  Bus Selector/1 -> x [m]/1  "<PositionX>"
  SELF/1 -> Bus Selector/1
  Gain/1 -> Demux2/1
  Demux2/1 -> rotx [deg]/1
  Demux2/2 -> roty [deg]/1
  Demux2/3 -> rotz [deg]/1
  compas converter/1(heading [deg]) -> heading [deg]/1
  Gain1/1 -> yaw rate [deg/s]/1

== system Demo_MostImportant_cs/BMW_X5_2/VISUColorRegion_Exterior_Mux ==
  RGB [-,-,-] : Inport
  Bus Creator : BusCreator  OutDataTypeStr=Bus: PRESCAN_COLOR_DATA  NonVirtualBus=on
  Constant : Constant  Value=255  OutDataTypeStr=uint8
  Data Type Conversion : DataTypeConversion  OutDataTypeStr=uint8
  Data Type Conversion1 : DataTypeConversion  OutDataTypeStr=uint8
  Data Type Conversion2 : DataTypeConversion  OutDataTypeStr=uint8
  Demux : Demux  Outputs=3
  ColorRegion : Outport  OutDataTypeStr=Bus: PRESCAN_COLOR_DATA  PortDimensions=1
  wires:
  Constant/1 -> Bus Creator/4  "A"
  Data Type Conversion2/1 -> Bus Creator/3  "B"
  Data Type Conversion1/1 -> Bus Creator/2  "G"
  Data Type Conversion/1 -> Bus Creator/1  "R"
  Demux/3 -> Data Type Conversion2/1  "B"
  Demux/2 -> Data Type Conversion1/1  "G"
  Demux/1 -> Data Type Conversion/1  "R"
  RGB [-,-,-]/1 -> Demux/1
  Bus Creator/1 -> ColorRegion/1

== system Demo_MostImportant_cs/BMW_X5_2/color_changing_logic ==
  Index_order : Inport
  Compare To Constant : simulink/Logic and Bit Operations/Compare To Constant  relop=<=  const=3  OutDataTypeStr=uint8  ZeroCross=off
  Multiport Switch : MultiPortSwitch  DataPortOrder=Zero-based contiguous  Inputs=4  zeroidx=on
  Product : Product  RndMeth=Zero
  TextureColor1 : Constant  Tag=TextureColor  Value="[255 0  0]"
  TextureColor2 : Constant  Tag=TextureColor  Value="[211  211  211]"
  TextureColor3 : Constant  Tag=TextureColor  Value=[255 128 0]
  TextureColor4 : Constant  Tag=TextureColor  Value=[255 255 55]
  RGB : Outport
  wires:
  TextureColor2/1 -> Multiport Switch/2  "L21"
  TextureColor1/1 -> Multiport Switch/3  "L21"
  TextureColor3/1 -> Multiport Switch/4
  Compare To Constant/1 -> Product/2
  Index_order/1 -> Product/1, Compare To Constant/1
  Product/1 -> Multiport Switch/1
  Multiport Switch/1 -> RGB/1  "L47"
  TextureColor4/1 -> Multiport Switch/5

== system Demo_MostImportant_cs/Citroen_C3_1/Dynamics_Empty ==
  note: For state mode 'Dynamic' positions
      | are not taken into account, as they
      | are computed by integrating velocity.
      | Click annotation for Help.
  Ground_{1..9} (9 alike) : Ground
  MuxState : Subsystem  Tag=mux/State  mask(Empty Dynamics State Block){positioningmode=on, TimeStep=1/20}
      mask prompts: positioningmode "Positioning Mode"; TimeStep "Auto Assigned: Time Step [s]"
      mask help:
      | Build the state of an actor based on user input.
      | The user can either use positioning mode or dynamics mode.
      | - When using positioning mode the position and orientation of the actor are set directly based on the input. Expected input is relative to the initial position and orientation of the actor. It's also possible to specify the velocity of the actor, though this input isn't used, only passed on.
      | - When using dynamics mode the position input is ignored. Expected input is velocity and orientation. The velocity is relative the current orientation of the actor, while orientation is relative to its initial orientation. The position of the actor is calculated based on the velocity and orientation given.
      settings: DeleteFcn=PreScanBlockDeleteFcn;
  STATE_Citroen_C3_1 : Subsystem  Tag=mux/StatePort  Priority=0  LoadFcn=load PrescanStateActuatorData  mask(PreScan Sink Block: State){x0=Demo_MostImportant_cs_d90e04aced6e68bf, y0=Demo_MostImportant_cs_90ff3a0811121d4c, z0=Demo_MostImportant_cs_0fd3352235f3d862, Roll0=Demo_MostImportant_cs_c34fad1f7dbabd44, Pitch0=Demo_MostImportant_cs_3bee97dace5a3f8a, Yaw0=Demo_MostImportant_cs_4a85c22e4a955f8e, TimeStep=1/20}
      mask prompts: x0 "Ini x-position VEHICLE wrt GLOBAL axis system [m]"; y0 "Ini y-position VEHICLE wrt GLOBAL axis system [m]"; z0 "Ini z-position VEHICLE wrt GLOBAL axis system [m]"; Roll0 "Ini roll-angle BODY wrt VEHICLE axis system [deg]"; Pitch0 "Ini pitch-angle BODY wrt VEHICLE axis system [deg]"; Yaw0 "Ini yaw-angle VEHICLE wrt GLOBAL axis system [deg]"; TimeStep "Auto-Assigned: Upload Period [s]"
      mask help:
      | The Actor State contains a vector signal of size (9x1), containing the following signals:
      |
      | -  Position                  (x,y,z)                                     [m]
      | -  Velocity                  (vx,vy,vz)                               [m/s]
      | -  Angles                    (Roll, Pitch, Yaw)                   [rad]
      |
      | The Actor state is defined in the global axis system.
      | The state is superponed on the Initial position defined in the GUI.
      |
      | For more information, please click Help.
      settings: DeleteFcn=PreScanBlockDeleteFcn;
      mask Help: eval('openHelp(222)')
      mask Display: image(imread('State.png'))
  State : Outport  Tag=outport/StateOutport  SampleTime=1/20
  wires:
  MuxState/1(state) -> STATE_Citroen_C3_1/1(State)
  STATE_Citroen_C3_1/1(StateBus) -> State/1
  Ground_1/1 -> MuxState/1(x [m])
  Ground_2/1 -> MuxState/2(y [m])
  Ground_3/1 -> MuxState/3(z [m])
  Ground_4/1 -> MuxState/4(dx [m/s])
  Ground_5/1 -> MuxState/5(dy [m/s])
  Ground_6/1 -> MuxState/6(dz [m/s])
  Ground_7/1 -> MuxState/7(R [rad])
  Ground_8/1 -> MuxState/8(P [rad])
  Ground_9/1 -> MuxState/9(Y [rad])

== system Demo_MostImportant_cs/Citroen_C3_1/SELF_Demux ==
  SELF : Inport  OutDataTypeStr=Bus: PRESCAN_SELFSENSORDATA
  Bus Selector : BusSelector  OutputSignals=PositionX,PositionY,PositionZ,OrientationRoll,OrientationPitch,OrientationYaw,Velocity,Yaw_rate,Lat,Long,Alt
  Demux2 : Demux  Outputs=3
  Gain : Gain  Gain=180/pi
  Gain1 : Gain  Gain=180/pi
  Vector Concatenate1 : Concatenate  NumInputs=3
  compas converter : Subsystem
  x [m] : Outport
  y [m] : Outport  Port=2
  z [m] : Outport  Port=3
  rotx [deg] : Outport  Port=4
  roty [deg] : Outport  Port=5
  rotz [deg] : Outport  Port=6
  GPS lat [deg] : Outport  Port=7
  GPS long [deg] : Outport  Port=8
  GPS alt [m] : Outport  Port=9
  velocity [m/s] : Outport  Port=10
  heading [deg] : Outport  Port=11
  yaw rate [deg/s] : Outport  Port=12
  wires:
  Bus Selector/11 -> GPS alt [m]/1  "<Alt>"
  Bus Selector/10 -> GPS long [deg]/1  "<Long>"
  Bus Selector/9 -> GPS lat [deg]/1  "<Lat>"
  Bus Selector/8 -> Gain1/1  "<Yaw_rate>"
  Bus Selector/7 -> velocity [m/s]/1  "<Velocity>"
  Bus Selector/6 -> compas converter/1(rotz [rad]), Vector Concatenate1/3  "<OrientationYaw>"
  Bus Selector/5 -> Vector Concatenate1/2  "<OrientationPitch>"
  Bus Selector/4 -> Vector Concatenate1/1  "<OrientationRoll>"
  Vector Concatenate1/1 -> Gain/1
  Bus Selector/3 -> z [m]/1  "<PositionZ>"
  Bus Selector/2 -> y [m]/1  "<PositionY>"
  Bus Selector/1 -> x [m]/1  "<PositionX>"
  SELF/1 -> Bus Selector/1
  Gain/1 -> Demux2/1
  Demux2/1 -> rotx [deg]/1
  Demux2/2 -> roty [deg]/1
  Demux2/3 -> rotz [deg]/1
  compas converter/1(heading [deg]) -> heading [deg]/1
  Gain1/1 -> yaw rate [deg/s]/1

== system Demo_MostImportant_cs/Citroen_C3_1/VISUColorRegion_Exterior_Mux ==
  RGB [-,-,-] : Inport
  Bus Creator : BusCreator  OutDataTypeStr=Bus: PRESCAN_COLOR_DATA  NonVirtualBus=on
  Constant : Constant  Value=255  OutDataTypeStr=uint8
  Data Type Conversion : DataTypeConversion  OutDataTypeStr=uint8
  Data Type Conversion1 : DataTypeConversion  OutDataTypeStr=uint8
  Data Type Conversion2 : DataTypeConversion  OutDataTypeStr=uint8
  Demux : Demux  Outputs=3
  ColorRegion : Outport  OutDataTypeStr=Bus: PRESCAN_COLOR_DATA  PortDimensions=1
  wires:
  Constant/1 -> Bus Creator/4  "A"
  Data Type Conversion2/1 -> Bus Creator/3  "B"
  Data Type Conversion1/1 -> Bus Creator/2  "G"
  Data Type Conversion/1 -> Bus Creator/1  "R"
  Demux/3 -> Data Type Conversion2/1  "B"
  Demux/2 -> Data Type Conversion1/1  "G"
  Demux/1 -> Data Type Conversion/1  "R"
  RGB [-,-,-]/1 -> Demux/1
  Bus Creator/1 -> ColorRegion/1

== system Demo_MostImportant_cs/Citroen_C3_1/color_changing_logic ==
  Index_order : Inport
  Compare To Constant : simulink/Logic and Bit Operations/Compare To Constant  relop=<=  const=3  OutDataTypeStr=uint8  ZeroCross=off
  Multiport Switch : MultiPortSwitch  DataPortOrder=Zero-based contiguous  Inputs=4  zeroidx=on
  Product : Product  RndMeth=Zero
  TextureColor1 : Constant  Tag=TextureColor  Value="[255 0  0]"
  TextureColor2 : Constant  Tag=TextureColor  Value="[211  211  211]"
  TextureColor3 : Constant  Tag=TextureColor  Value=[255 128 0]
  TextureColor4 : Constant  Tag=TextureColor  Value=[255 255 55]
  RGB : Outport
  wires:
  TextureColor2/1 -> Multiport Switch/2  "L21"
  TextureColor1/1 -> Multiport Switch/3  "L21"
  TextureColor3/1 -> Multiport Switch/4
  Compare To Constant/1 -> Product/2
  Index_order/1 -> Product/1, Compare To Constant/1
  Product/1 -> Multiport Switch/1
  Multiport Switch/1 -> RGB/1  "L47"
  TextureColor4/1 -> Multiport Switch/5
